simulink model "control_PID_model"  (R2015a)
settings: Solver=ode8  StartTime=0.0  StopTime=10.0  FixedStep=0.01  RelTol=1e-3
values from neighbouring files (symbols this model uses):
  gear_ratio = 25    [experiment1.mat]    (also in experiment2.mat; experiment3.mat; experiment4.mat; friction_ident.mat)
  max_voltage = 13.3    [experiment1.mat]    (also in experiment2.mat; experiment3.mat; experiment4.mat; friction_ident.mat)
libraries: simulink x1
settings Model: Creator=Student  LastModifiedBy=Student

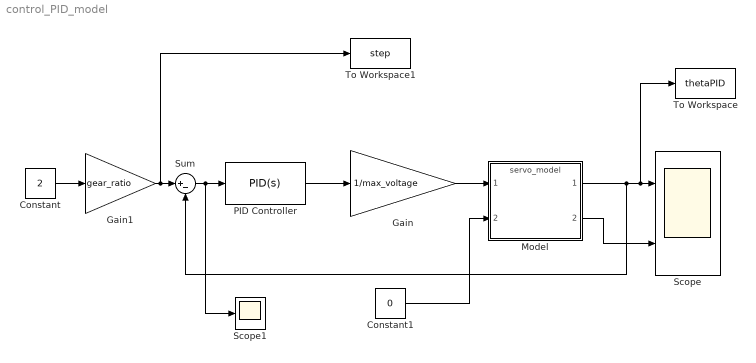
== system control_PID_model ==
  Constant : Constant  Value=2
  Constant1 : Constant  Value=0
  Gain : Gain  Gain=1/max_voltage
  Gain1 : Gain  Gain=gear_ratio
  Model : ModelReference  ModelNameDialog=servo_model.slx  SimulationMode=Normal  ModelReferenceVersion=1.27  CopyOfModelName=servo_model.slx  DefaultDataLogging=on
  PID Controller : simulink/Continuous/PID Controller  Controller=PID  TimeDomain=Continuous-time  SampleTime=-1  IntegratorMethod=Forward Euler  FilterMethod=Forward Euler  Form=Parallel  UseFilter=on  ControllerParametersSource=internal  P=1.28114968885398  I=0.174066106483071  D=0.923302107057059  N=139.71964045646  InitialConditionSource=internal  InitialConditionForIntegrator=0  InitialConditionForFilter=0  ExternalReset=none  LimitOutput=off  UpperSaturationLimit=inf  LowerSaturationLimit=-inf  LinearizeAsGain=on  AntiWindupMode=none  Kb=1  TrackingMode=off  Kt=1  PParamMin=[]  PParamMax=[]  IParamMin=[]  IParamMax=[]  DParamMin=[]  DParamMax=[]  NParamMin=[]  NParamMax=[]  KbParamMin=[]  KbParamMax=[]  KtParamMin=[]  KtParamMax=[]  POutMin=[]  POutMax=[]  IOutMin=[]  IOutMax=[]  DOutMin=[]  DOutMax=[]  NOutMin=[]  NOutMax=[]  KbOutMin=[]  KbOutMax=[]  KtOutMin=[]  KtOutMax=[]  IntegratorOutMin=[]  IntegratorOutMax=[]  FilterOutMin=[]  FilterOutMax=[]  SumOutMin=[]  SumOutMax=[]  SumI1OutMin=[]  SumI1OutMax=[]  SumI2OutMin=[]  SumI2OutMax=[]  SumI3OutMin=[]  SumI3OutMax=[]  SumDOutMin=[]  SumDOutMax=[]  SaturationOutMin=[]  SaturationOutMax=[]  IntegratorContinuousStateAttributes=''  IntegratorStateMustResolveToSignalObject=off  IntegratorRTWStateStorageClass=Auto  FilterContinuousStateAttributes=''  FilterStateMustResolveToSignalObject=off  FilterRTWStateStorageClass=Auto  DifferentiatorICPrevScaledInput=0  DifferentiatorOutMin=[]  DifferentiatorOutMax=[]
  Scope : Scope  NumInputPorts=2
      settings: YMin=-5~-5  YMax=5~5
  Scope1 : Scope
  Sum : Sum  Inputs=|+-
  To Workspace : ToWorkspace  VariableName=thetaPID  SampleTime=-1
  To Workspace1 : ToWorkspace  VariableName=step  SampleTime=-1
  wires:
  Gain/1 -> Model/1
  Model/1 -> To Workspace/1, Scope/1, Sum/2
  Sum/1 -> Scope1/1, PID Controller/1
  Constant/1 -> Gain1/1
  PID Controller/1 -> Gain/1
  Model/2 -> Scope/2
  Gain1/1 -> To Workspace1/1, Sum/1
  Constant1/1 -> Model/2
